simulink model "ex_28_model_f1"  (R2014a)
settings: Solver=ode45  StartTime=0.0  StopTime=0.25  RelTol=1e-3
values from neighbouring files (symbols this model uses):
  ki = ((Kp*(K^2+a*R)) / (J*R))    (= 1.0404)    [ex_28_init.m]
  Kp = -1/(y/x)    (= 0.051)    [ex_28_init.m]    (also in ex_28_plots.m = Kp*10)
  Kp0 = Kp    (= 0.051)    [ex_28_init.m]
  x = -(1/J) * (a + (K^2/R))    (= -20.4)    [ex_28_init.m]
  y = (K/(J*R))    (= 400)    [ex_28_init.m]
  z = -(1/J)    (= -4000)    [ex_28_init.m]
settings Model: Creator=Nino  LastModifiedBy=Nino

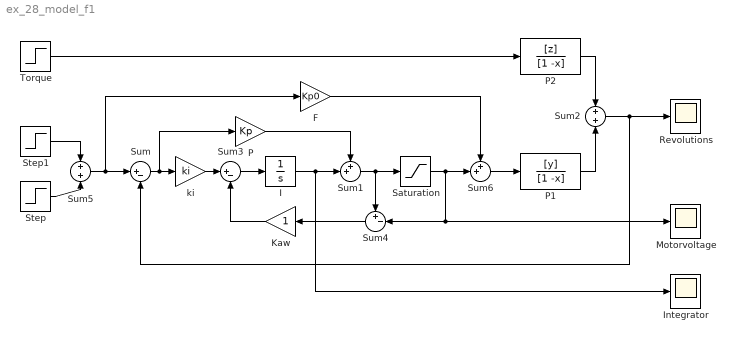
== system ex_28_model_f1 ==
  F : Gain  Gain=Kp0
  I : Integrator
  Integrator : Scope
      settings: YMin=0.9989  YMax=0.9999  SaveName=Integrator
  Kaw : Gain
  "Motorvoltage " : Scope
      settings: YMin=0.9989  YMax=0.9999  SaveName=Motorvoltage
  P : Gain  Gain=Kp
  P1 : TransferFcn  Numerator=[y]  Denominator=[1 -x]
  P2 : TransferFcn  Numerator=[z]  Denominator=[1 -x]
  Revolutions : Scope
      settings: YMin=0.9989  YMax=0.9999  SaveName=Revolutions
  Saturation : Saturate  UpperLimit=10  LowerLimit=-10  LinearizeAsGain=off
  Step : Step  Time=10000  After=0  SampleTime=0
  Step1 : Step  Time=0.1  Before=50  After=100  SampleTime=0
  Sum : Sum  Inputs=|+-
  Sum1 : Sum  Inputs=++|
  Sum2 : Sum  Inputs=+|+
  Sum3 : Sum  Inputs=|+-
  Sum4 : Sum  Inputs=+-|
  Sum5 : Sum  Inputs=+|+
  Sum6 : Sum  Inputs=++|
  Torque : Step  Time=100  After=0.5  SampleTime=0
  ki : Gain  Gain=ki
  wires:
  Torque/1 -> P2/1
  P2/1 -> Sum2/1
  Sum2/1 -> Sum/2, Revolutions/1
  Sum5/1 -> F/1, Sum/1
  Sum/1 -> P/1, ki/1
  P/1 -> Sum1/1
  I/1 -> Integrator/1, Sum1/2
  P1/1 -> Sum2/2
  Saturation/1 -> Sum6/2, Sum4/2, "Motorvoltage "/1
  Sum1/1 -> Saturation/1, Sum4/1
  ki/1 -> Sum3/1
  Sum3/1 -> I/1
  Sum4/1 -> Kaw/1
  Kaw/1 -> Sum3/2
  Step1/1 -> Sum5/1
  Step/1 -> Sum5/2
  Sum6/1 -> P1/1
  F/1 -> Sum6/1
